simulink model "exp1_PI_v2017a"  (R2017a)
settings: Solver=VariableStepAuto  StartTime=0.0  StopTime=10.0  RelTol=1e-3
settings Model: Creator=ansshuman  LastModifiedBy=ansshuman
settings DataIOCC: ReturnWorkspaceOutputs=on
settings SFSimCC: SimUseLocalCustomCode=on
settings RTWCC: RTWUseLocalCustomCode=on

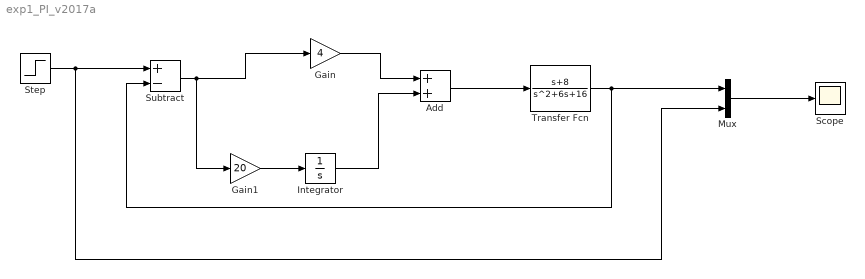
== system exp1_PI_v2017a ==
  Add : Sum
  Gain : Gain  Gain=4
  Gain1 : Gain  Gain=20
  Integrator : Integrator
  Mux : Mux  Inputs=2
  Scope : Scope
  Step : Step  SampleTime=0
  Subtract : Sum  Inputs=+-
  Transfer Fcn : TransferFcn  Numerator=[1, 8]  Denominator=[1, 6, 16]
  wires:
  Subtract/1 -> Gain1/1, Gain/1
  Gain1/1 -> Integrator/1
  Integrator/1 -> Add/2
  Gain/1 -> Add/1
  Add/1 -> Transfer Fcn/1
  Transfer Fcn/1 -> Subtract/2, Mux/1
  Step/1 -> Mux/2, Subtract/1
  Mux/1 -> Scope/1
